simulink model "DISCON_NREL5MW_WaveFF"  (R2023b)
settings: Solver=ode1  StartTime=0.0  StopTime=inf  FixedStep=Control.TimeStep  RelTol=1e-3
InitFcn:
  | % General parameters
  | DT=0.0565685;
  | Control.TimeStep=DT;
  | gb=97;
settings Model: Creator=evansolingen  LastModifiedBy=rmojal
settings SolverCC: AlgebraicLoopSolver=TrustRegion
settings DataIOCC: LimitDataPoints=on  SaveFormat=Array  SignalLoggingSaveFormat=ModelDataLogs  SaveOutput=off  SignalLogging=off  SaveTime=off  ReturnWorkspaceOutputs=off
settings OptimizationCC: ExpressionDepthLimit=2147483647  LifeSpan=inf
settings DebuggingCC: UnderspecifiedInitializationDetection=Classic  MergeDetectMultiDrivingBlocksExec=none  SolverPrmCheckMsg=warning  MultiTaskDSMMsg=warning  MultiTaskCondExecSysMsg=none  FcnCallInpInsideContextMsg=warning  UnconnectedInputMsg=warning  UnconnectedOutputMsg=warning  UnconnectedLineMsg=warning  AllowSymbolicDim=off  StateNameClashWarn=warning  SFUnexpectedBacktrackingDiag=warning  SFNoUnconditionalDefaultTransitionDiag=warning  SFExecutionAtInitializationDiag=none  ArithmeticOperatorsInVariantConditions=warning
settings HardwareCC: ProdBitPerPointer=32  ProdBitPerSizeT=32  ProdBitPerPtrDiffT=32  ProdLargestAtomicFloat=None  ProdIntDivRoundTo=Undefined  ProdWordSize=32  ProdHWDeviceType=32-bit Generic  TargetEndianess=LittleEndian
settings ModelReferenceCC: UpdateModelReferenceTargets=Force  EnableRefExpFcnMdlSchedulingChecks=on  PropagateSignalLabelsOutOfModel=off
settings SFSimCC: SimUseLocalCustomCode=off  SimParseCustomCode=off  CustomCodeUndefinedFunction=UseInterfaceOnly
settings RTWCC: Description=DISCON DLL Target (for use with GH BLADED)  SystemTargetFile=discon.tlc  TemplateMakefile=discon.tmf  RTWUseLocalCustomCode=off
settings CodeAppCC: StateflowObjectComments=on
settings GRTTargetCC: TargetLangStandard=C89/C90 (ANSI)  CombineOutputUpdateFcns=off  GRTInterface=on  UseToolchainInfoCompliant=off  ExtModeMexFile=noextcomm
settings ConfigComp: CovMetricSettings=dw  CovSaveCumulativeToWorkspaceVar=on  CovSaveSingleToWorkspaceVar=on  CovExternalEMLEnable=off

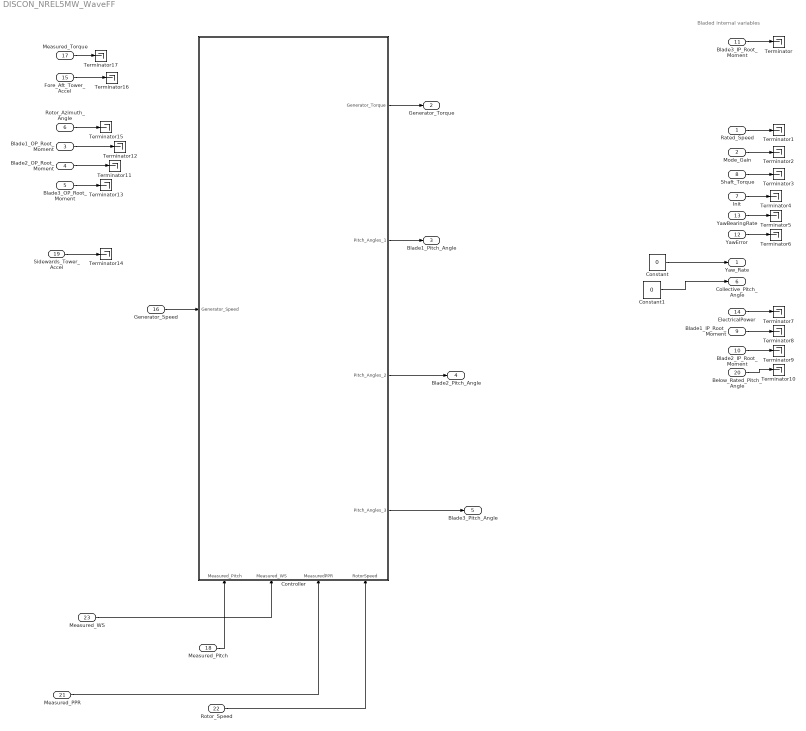
== system DISCON_NREL5MW_WaveFF ==
  note: Bladed internal variables
  Rated_Speed : Inport  PortDimensions=1
  Mode_Gain : Inport  Port=2  PortDimensions=1
  Blade1_OP_Root_Moment : Inport  Port=3  PortDimensions=1
  Blade2_OP_Root_Moment : Inport  Port=4  PortDimensions=1
  Blade3_OP_Root_Moment : Inport  Port=5  PortDimensions=1
  Rotor_Azimuth_Angle : Inport  Port=6  PortDimensions=1
  Init : Inport  Port=7  PortDimensions=1
  Shaft_Torque : Inport  Port=8  PortDimensions=1
  Blade1_IP_Root_Moment : Inport  Port=9  PortDimensions=1
  Blade2_IP_Root_Moment : Inport  Port=10  PortDimensions=1
  Blade3_IP_Root_Moment : Inport  Port=11  PortDimensions=1
  YawError : Inport  Port=12  PortDimensions=1
  YawBearingRate : Inport  Port=13  PortDimensions=1
  ElectricalPower : Inport  Port=14  PortDimensions=1
  Fore_Aft_Tower_Accel : Inport  Port=15  PortDimensions=1
  Generator_Speed : Inport  Port=16  PortDimensions=1
  Measured_Torque : Inport  Port=17  PortDimensions=1
  Measured_Pitch : Inport  Port=18  PortDimensions=1
  Sidewards_Tower_Accel : Inport  Port=19  PortDimensions=1
  Below_Rated_Pitch_Angle : Inport  Port=20  PortDimensions=1
  Measured_PPR : Inport  Port=21  PortDimensions=1
  Rotor_Speed : Inport  Port=22  PortDimensions=1
  Measured_WS : Inport  Port=23  PortDimensions=1
  Constant : Constant  Value=0
  Constant1 : Constant  Value=0
  Controller : Subsystem
      settings: PortSchema="{\"entries\":[{\"content\":{\"sides\":[{\"content\":{\"connectorIds\":[\"In1\"]},\"type\":\"ConnectorPlacement.EquallySpacedRectSide\",\"uuid\":\"5eea0745-7772-402e-b13d-af5dbe336d94\"},{\"content\":{\"connectorIds\":[\"Out1\",\"Out2\",\"Out3\",\"Out4\"],\"side\":\"RIGHT\"},\"type\":\"ConnectorPlacement.EquallySpacedRectSide\",\"uuid\":\"fe86a02a-1155-422e-9e4f-83d0aa3f1667\"},{\"content\":{\"side\":\"TOP\"},\"type\":\"ConnectorPlacement.EquallySpacedRectSide\",\"uuid\":\"d4d110c7-6a91-4408-ae2d-caf3a921c34f\"},{\"content\":{\"connectorIds\":[\"In2\",\"In3\",\"In4\",\"In5\"],\"side\":\"BOTTOM\"},\"type\":\"ConnectorPlacement.EquallySpacedRectSide\",\"uuid\":\"623fd245-908b-43aa-8a72-77a4c8000db8\"}]},\"type\":\"ConnectorPlacement.EquallySpacedConnector\",\"uuid\":\"2baef728-2889-41b2-b1a7-ad06cd068c9a\"}],\"packageUris\":[\"http://schema.mathworks.com/mf0/Connector/R2020b\"],\"version\":\"1.0\"}"
  Terminator{,1..17} (18 alike) : Terminator
  Yaw_Rate : Outport  PortDimensions=1  VectorParamsAs1DForOutWhenUnconnected=off
  Generator_Torque : Outport  Port=2  PortDimensions=1  VectorParamsAs1DForOutWhenUnconnected=off
  Blade1_Pitch_Angle : Outport  Port=3  PortDimensions=1  VectorParamsAs1DForOutWhenUnconnected=off
  Blade2_Pitch_Angle : Outport  Port=4  PortDimensions=1  VectorParamsAs1DForOutWhenUnconnected=off
  Blade3_Pitch_Angle : Outport  Port=5  PortDimensions=1  VectorParamsAs1DForOutWhenUnconnected=off
  Collective_Pitch_Angle : Outport  Port=6  PortDimensions=1  VectorParamsAs1DForOutWhenUnconnected=off
  wires:
  Generator_Speed/1 -> Controller/1(Generator_Speed)
  Controller/1(Generator_Torque) -> Generator_Torque/1
  Controller/2(Pitch_Angles_1) -> Blade1_Pitch_Angle/1
  Controller/3(Pitch_Angles_2) -> Blade2_Pitch_Angle/1
  Controller/4(Pitch_Angles_3) -> Blade3_Pitch_Angle/1
  Measured_PPR/1 -> Controller/4(MeasuredPPR)
  Rotor_Speed/1 -> Controller/5(RotorSpeed)
  Measured_WS/1 -> Controller/3(Measured_WS)
  Measured_Pitch/1 -> Controller/2(Measured_Pitch)
  Blade3_IP_Root_Moment/1 -> Terminator/1
  Rated_Speed/1 -> Terminator1/1
  Mode_Gain/1 -> Terminator2/1
  Shaft_Torque/1 -> Terminator3/1
  Init/1 -> Terminator4/1
  YawBearingRate/1 -> Terminator5/1
  YawError/1 -> Terminator6/1
  ElectricalPower/1 -> Terminator7/1
  Blade1_IP_Root_Moment/1 -> Terminator8/1
  Blade2_IP_Root_Moment/1 -> Terminator9/1
  Below_Rated_Pitch_Angle/1 -> Terminator10/1
  Blade1_OP_Root_Moment/1 -> Terminator12/1
  Blade2_OP_Root_Moment/1 -> Terminator11/1
  Blade3_OP_Root_Moment/1 -> Terminator13/1
  Sidewards_Tower_Accel/1 -> Terminator14/1
  Rotor_Azimuth_Angle/1 -> Terminator15/1
  Fore_Aft_Tower_Accel/1 -> Terminator16/1
  Measured_Torque/1 -> Terminator17/1
  Constant/1 -> Yaw_Rate/1
  Constant1/1 -> Collective_Pitch_Angle/1

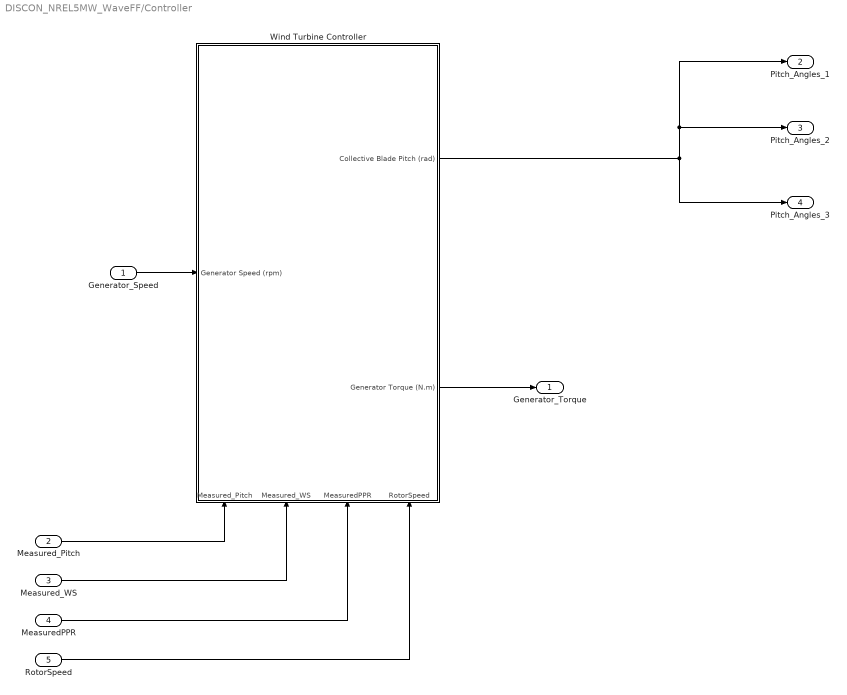
== system DISCON_NREL5MW_WaveFF/Controller ==
  Generator_Speed : Inport
  Measured_Pitch : Inport  Port=2
  Measured_WS : Inport  Port=3
  MeasuredPPR : Inport  Port=4
  RotorSpeed : Inport  Port=5
  Wind Turbine Controller : Subsystem
      settings: PortSchema="{\"entries\":[{\"content\":{\"sides\":[{\"content\":{\"connectorIds\":[\"In1\"]},\"type\":\"ConnectorPlacement.EquallySpacedRectSide\",\"uuid\":\"60e180a6-f3d9-41ac-b258-85164fa97132\"},{\"content\":{\"connectorIds\":[\"Out1\",\"Out2\"],\"side\":\"RIGHT\"},\"type\":\"ConnectorPlacement.EquallySpacedRectSide\",\"uuid\":\"a424f4c7-ff92-4106-8929-f61da2bed5ce\"},{\"content\":{\"side\":\"TOP\"},\"type\":\"ConnectorPlacement.EquallySpacedRectSide\",\"uuid\":\"4507b62c-853f-4db2-8819-247504761e25\"},{\"content\":{\"connectorIds\":[\"In2\",\"In3\",\"In4\",\"In5\"],\"side\":\"BOTTOM\"},\"type\":\"ConnectorPlacement.EquallySpacedRectSide\",\"uuid\":\"74ae92db-9457-4ead-8989-dbd06da1e1bc\"}]},\"type\":\"ConnectorPlacement.EquallySpacedConnector\",\"uuid\":\"890c16f4-d26b-446d-8a10-315b447bcdfe\"}],\"packageUris\":[\"http://schema.mathworks.com/mf0/Connector/R2020b\"],\"version\":\"1.0\"}"
  Generator_Torque : Outport  VectorParamsAs1DForOutWhenUnconnected=off
  Pitch_Angles_1 : Outport  Port=2  PortDimensions=1  VectorParamsAs1DForOutWhenUnconnected=off
  Pitch_Angles_2 : Outport  Port=3  PortDimensions=1  VectorParamsAs1DForOutWhenUnconnected=off
  Pitch_Angles_3 : Outport  Port=4  PortDimensions=1  VectorParamsAs1DForOutWhenUnconnected=off
  wires:
  Wind Turbine Controller/2(Generator Torque (N.m)) -> Generator_Torque/1
  Generator_Speed/1 -> Wind Turbine Controller/1(Generator Speed (rpm))
  Wind Turbine Controller/1(" Collective Blade Pitch (rad)") -> Pitch_Angles_1/1, Pitch_Angles_2/1, Pitch_Angles_3/1
  MeasuredPPR/1 -> Wind Turbine Controller/4(MeasuredPPR)
  RotorSpeed/1 -> Wind Turbine Controller/5(RotorSpeed)
  Measured_Pitch/1 -> Wind Turbine Controller/2(Measured_Pitch)
  Measured_WS/1 -> Wind Turbine Controller/3(Measured_WS)

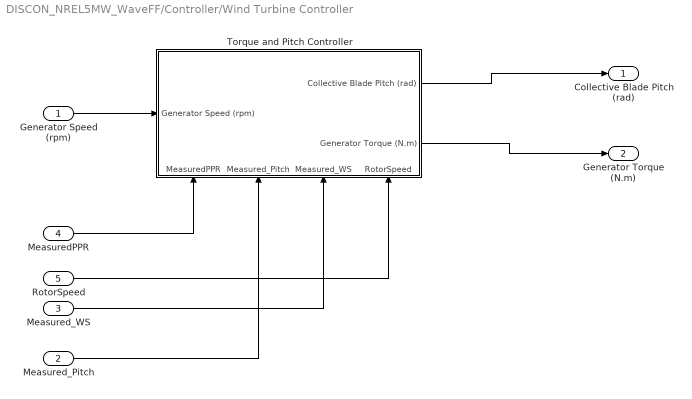
== system DISCON_NREL5MW_WaveFF/Controller/Wind Turbine Controller ==
  Generator Speed (rpm) : Inport
  Measured_Pitch : Inport  Port=2
  Measured_WS : Inport  Port=3
  MeasuredPPR : Inport  Port=4
  RotorSpeed : Inport  Port=5
  Torque and Pitch Controller : Subsystem
      settings: PortSchema="{\"entries\":[{\"content\":{\"sides\":[{\"content\":{\"connectorIds\":[\"In1\"]},\"type\":\"ConnectorPlacement.EquallySpacedRectSide\",\"uuid\":\"41f078d3-b4c7-4436-8efb-2933835bf469\"},{\"content\":{\"connectorIds\":[\"Out1\",\"Out2\"],\"side\":\"RIGHT\"},\"type\":\"ConnectorPlacement.EquallySpacedRectSide\",\"uuid\":\"44137c6d-4d2f-4b5d-90b4-72e44e418c3d\"},{\"content\":{\"side\":\"TOP\"},\"type\":\"ConnectorPlacement.EquallySpacedRectSide\",\"uuid\":\"9ef615e9-cc73-41b1-8842-e294b4be6557\"},{\"content\":{\"connectorIds\":[\"In2\",\"In3\",\"In4\",\"In5\"],\"side\":\"BOTTOM\"},\"type\":\"ConnectorPlacement.EquallySpacedRectSide\",\"uuid\":\"69c559ae-5e90-48b5-8bb5-f3e725c72204\"}]},\"type\":\"ConnectorPlacement.EquallySpacedConnector\",\"uuid\":\"6facd867-2bfd-4329-8099-ae66f4e4d363\"}],\"packageUris\":[\"http://schema.mathworks.com/mf0/Connector/R2020b\"],\"version\":\"1.0\"}"
  " Collective Blade Pitch (rad)" : Outport
  Generator Torque (N.m) : Outport  Port=2
  wires:
  Generator Speed (rpm)/1 -> Torque and Pitch Controller/1(Generator Speed (rpm))
  Torque and Pitch Controller/2(Generator Torque (N.m)) -> Generator Torque (N.m)/1
  Torque and Pitch Controller/1(" Collective Blade Pitch (rad)") -> " Collective Blade Pitch (rad)"/1
  MeasuredPPR/1 -> Torque and Pitch Controller/2(MeasuredPPR)
  RotorSpeed/1 -> Torque and Pitch Controller/5(RotorSpeed)
  Measured_WS/1 -> Torque and Pitch Controller/4(Measured_WS)
  Measured_Pitch/1 -> Torque and Pitch Controller/3(Measured_Pitch)

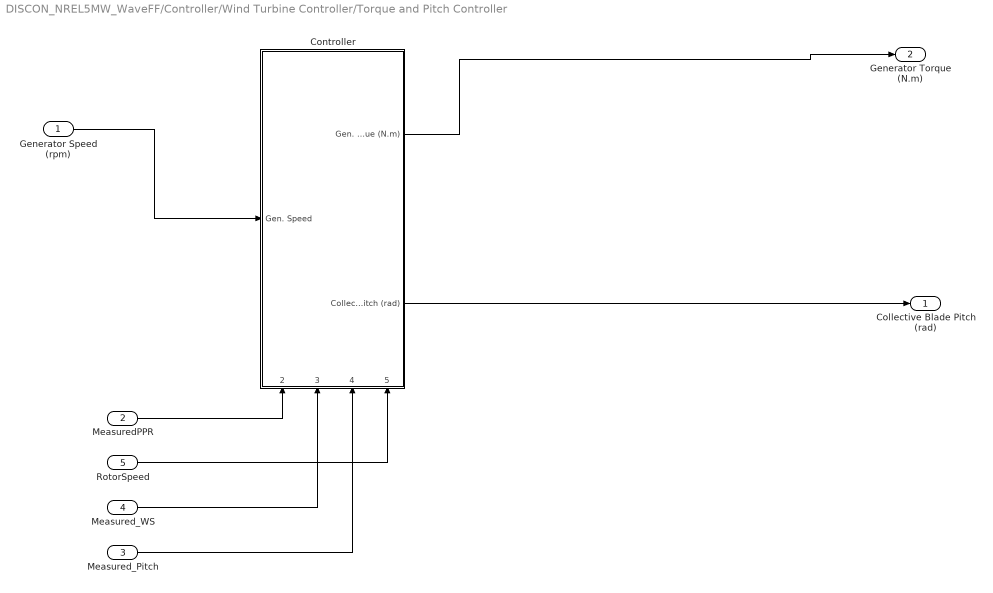
== system DISCON_NREL5MW_WaveFF/Controller/Wind Turbine Controller/Torque and Pitch Controller ==
  Generator Speed (rpm) : Inport
  MeasuredPPR : Inport  Port=2
  Measured_Pitch : Inport  Port=3
  Measured_WS : Inport  Port=4
  RotorSpeed : Inport  Port=5
  Controller : Subsystem
      settings: PortSchema="{\"entries\":[{\"content\":{\"sides\":[{\"content\":{\"connectorIds\":[\"In1\"]},\"type\":\"ConnectorPlacement.EquallySpacedRectSide\",\"uuid\":\"059e71ba-ba04-4257-a8ec-4ba8011e6b7c\"},{\"content\":{\"connectorIds\":[\"Out1\",\"Out2\"],\"side\":\"RIGHT\"},\"type\":\"ConnectorPlacement.EquallySpacedRectSide\",\"uuid\":\"7728fccf-4111-43b7-a29b-3c8202db8d59\"},{\"content\":{\"side\":\"TOP\"},\"type\":\"ConnectorPlacement.EquallySpacedRectSide\",\"uuid\":\"5cd4fe85-95f9-47fb-ae2b-ff437f261722\"},{\"content\":{\"connectorIds\":[\"In2\",\"In3\",\"In4\",\"In5\"],\"side\":\"BOTTOM\"},\"type\":\"ConnectorPlacement.EquallySpacedRectSide\",\"uuid\":\"633850b7-9343-4aec-ae47-23a99e859344\"}]},\"type\":\"ConnectorPlacement.EquallySpacedConnector\",\"uuid\":\"ea1a022b-361d-480f-a696-27bf9479e3d4\"}],\"packageUris\":[\"http://schema.mathworks.com/mf0/Connector/R2020b\"],\"version\":\"1.0\"}"
  " Collective Blade Pitch (rad)" : Outport
  Generator Torque (N.m) : Outport  Port=2
  wires:
  Controller/1(Gen. Torque (N.m)) -> Generator Torque (N.m)/1
  Generator Speed (rpm)/1 -> Controller/1(Gen. Speed)
  Controller/2(Collective Blade Pitch (rad)) -> " Collective Blade Pitch (rad)"/1
  MeasuredPPR/1 -> Controller/2(Measured_PPR)
  RotorSpeed/1 -> Controller/5(RotorSpeed)
  Measured_WS/1 -> Controller/3(Measured_WS)
  Measured_Pitch/1 -> Controller/4(Measured_Pitch)

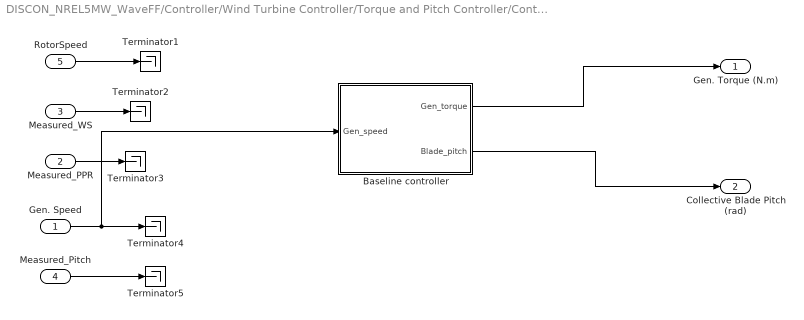
== system DISCON_NREL5MW_WaveFF/Controller/Wind Turbine Controller/Torque and Pitch Controller/Controller ==
  Gen. Speed : Inport
  Measured_PPR : Inport  Port=2
  Measured_WS : Inport  Port=3
  Measured_Pitch : Inport  Port=4
  RotorSpeed : Inport  Port=5
  Baseline controller : Subsystem
  Terminator{1..5} (5 alike) : Terminator
  Gen. Torque (N.m) : Outport
  Collective Blade Pitch (rad) : Outport  Port=2
  wires:
  RotorSpeed/1 -> Terminator1/1
  Measured_WS/1 -> Terminator2/1
  Measured_PPR/1 -> Terminator3/1
  Gen. Speed/1 -> Baseline controller/1(Gen_speed), Terminator4/1
  Measured_Pitch/1 -> Terminator5/1
  Baseline controller/1(Gen_torque) -> Gen. Torque (N.m)/1
  Baseline controller/2(Blade_pitch) -> Collective Blade Pitch (rad)/1

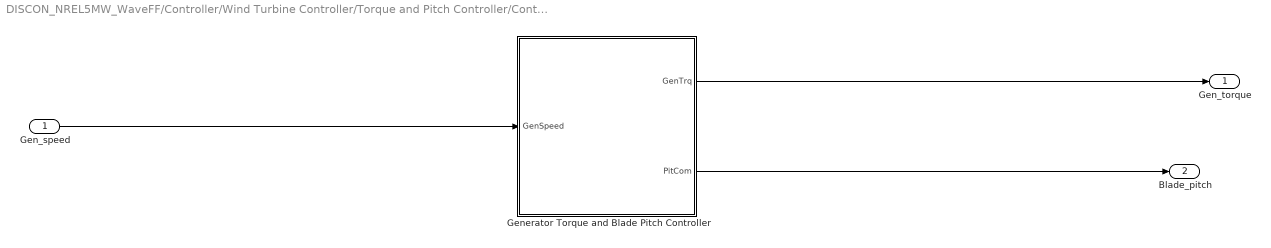
== system DISCON_NREL5MW_WaveFF/Controller/Wind Turbine Controller/Torque and Pitch Controller/Controller/Baseline controller ==
  Gen_speed : Inport
  Generator Torque and Blade Pitch Controller : MATLAB Function  TreatAsAtomicUnit=on
  Gen_torque : Outport
  Blade_pitch : Outport  Port=2
  wires:
  Generator Torque and Blade Pitch Controller/2(PitCom) -> Blade_pitch/1
  Gen_speed/1 -> Generator Torque and Blade Pitch Controller/1(GenSpeed)
  Generator Torque and Blade Pitch Controller/1(GenTrq) -> Gen_torque/1

== matlab function DISCON_NREL5MW_WaveFF/Controller/Wind Turbine Controller/Torque and Pitch Controller/Controller/Baseline controller/Generator Torque and Blade Pitch Controller ==
  data: GenTrq output; GenSpeed input; PitCom output; Control parameter
function [GenTrq, PitCom] = Controller(GenSpeed, Control)

%% Definition of the variables used in the script
% LPF_CornerFreq: Corner frequency (-3dB point) in the recursive, single-pole, low-pass filter, rad/s. -- chosen to be 1/4 the blade edgewise natural frequency ( 1/4 of approx. 1Hz = 0.25Hz = 1.570796rad/s)
% TimeStep      : Simulation time step (s)
% PC_DT         : Communication interval for pitch  controller, sec.
% PC_KI         : Integral gain for pitch controller at rated pitch (zero), (-).
% PC_KK         : Pitch angle where the the derivative of the aerodynamic power w.r.t. pitch has increased by a factor of two relative to the derivative at rated pitch (zero), rad.
% PC_KP         : Proportional gain for pitch controller at rated pitch (zero), sec.
% PC_MaxPit     : Maximum pitch setting in pitch controller, rad.
% PC_MaxRat     : Maximum pitch  rate (in absolute value) in pitch  controller, rad/s.
% PC_MinPit     : Minimum pitch setting in pitch controller, rad.
% PC_RefSpd     : Desired (reference) HSS speed for pitch controller, rad/s.
% PitCom        : Commanded pitch of each blade the last time the controller was called, rad.
% PitComI       : Integral term of command pitch, rad.
% PitComP       : Proportional term of command pitch, rad.
% PitComT       : Total command pitch based on the sum of the proportional and integral terms, rad.
% PitRate       : Pitch rates of each blade based on the current pitch angles and current pitch command, rad/s.
% SpdErr        : Current speed error, rad/s.
% TrqRate       : Torque rate based on the current and last torque commands, N-m/s.
% VS_CtInSp     : Transitional generator speed (HSS side) between regions 1 and 1 1/2, rad/s.
% VS_DT         : Communication interval for torque controller, sec.
% VS_MaxRat     : Maximum torque rate (in absolute value) in torque controller, N-m/s.
% VS_MaxTq      : Maximum generator torque in Region 3 (HSS side), N-m. -- chosen to be 10% above VS_RtTq = 43.09355kNm
% VS_Rgn2K      : Generator torque constant in Region 2 (HSS side), N-m/(rad/s)^2.
% VS_Rgn2Sp     : Transitional generator speed (HSS side) between regions 1 1/2 and 2, rad/s.
% VS_Rgn3MP     : Minimum pitch angle at which the torque is computed as if we are in region 3 regardless of the generator speed, rad. -- chosen to be 1.0 degree above PC_MinPit
% VS_RtGnSp     : Rated generator speed (HSS side), rad/s. -- chosen to be 99% of PC_RefSpd
% VS_RtPwr      : Rated generator generator power in Region 3, Watts. -- chosen to be 5MW divided by the electrical generator efficiency of 94.4%
% VS_Slope15    : Torque/speed slope of region 1 1/2 cut-in torque ramp , N-m/(rad/s).
% VS_Slope25    : Torque/speed slope of region 2 1/2 induction generator, N-m/(rad/s).
% VS_SlPc       : Rated generator slip percentage in Region 2 1/2, %.
% VS_SySp       : Synchronous speed of region 2 1/2 induction generator, rad/s.
% VS_TrGnSp     : Transitional generator speed (HSS side) between regions 2 and 2 1/2, rad/s.

% Note, each of the above variables is preceeded by the structure and the
% field where they are defined. That structure is called Control, and is
% composed of 4 field, namely, TimeStep, Filters, Torque and Pitch. 

%% Define the persistent variables in the function
persistent GenSpdFilt PitCommand GK SpdErrInt LastGenTorque 

%% Determine some torque control parameters not specified directly
VS_SySp       = Control.Torque.VS_RtGnSp/( 1.0 +  0.01*Control.Torque.VS_SlPc );                                                                         % Synchronous speed of region 2 1/2 induction generator, rad/s.
VS_Slope15    = (Control.Torque.VS_Rgn2K*Control.Torque.VS_Rgn2Sp*Control.Torque.VS_Rgn2Sp )/( Control.Torque.VS_Rgn2Sp - Control.Torque.VS_CtInSp );   % Torque/speed slope of region 1 1/2 cut-in torque ramp , N-m/(rad/s).
VS_Slope25    = ( Control.Torque.VS_RtPwr/Control.Pitch.PC_RefSpd           )/( Control.Torque.VS_RtGnSp - VS_SySp   );                                  % Torque/speed slope of region 2 1/2 induction generator , N-m/(rad/s).

if ( Control.Torque.VS_Rgn2K == 0.0 )
    VS_TrGnSp = VS_SySp;                                           % TRUE, if the torque in Region 2 is flat, and thus, the denominator in the ELSE condition is zero
else
    VS_TrGnSp = ( VS_Slope25 - sqrt( VS_Slope25*( VS_Slope25 - 4.0*Control.Torque.VS_Rgn2K*VS_SySp ) ) )/( 2.0*Control.Torque.VS_Rgn2K );
end

%% Initialize Saved Variables 
if isempty(GenSpdFilt)
    GenSpdFilt = GenSpeed;                                         % This will ensure that generator speed filter will use the initial value of the generator speed on the first pass                
    PitCommand = Control.Pitch.PC_MinPit;                          % This will ensure that the variable speed controller picks the correct control region and the pitch controller picks the correct gain on the first call
    GK         = 1.0/( 1.0 + PitCommand/Control.Pitch.PC_KK );     % This will ensure that the pitch angle is unchanged if the initial SpdErr is zero
    SpdErrInt  = PitCommand/( GK*Control.Pitch.PC_KI );            % This will ensure that the pitch angle is unchanged if the initial SpdErr is zero    
end

%% ============================= Filtering ============================= %%
% Filter the HSS (generator) speed measurement
% NOTE: This is a very simple recursive, single-pole, low-pass filter with exponential smoothing.
Alpha         = exp( -Control.TimeStep * Control.Filters.LPF_CornerFreq );

% Apply the Filter
GenSpeedF = ( 1.0 - Alpha )*GenSpeed + Alpha * GenSpdFilt;

% Update the persistent variable GenSpdFilt (This is to store the value of the presistent variable to be e used in the next time step)
GenSpdFilt = GenSpeedF;
     
%% =================== Variable-Speed Torque Control =================== %%
% Compute the generator torque, which depends on which region we are in:
if(GenSpeedF >= Control.Torque.VS_RtGnSp)||( PitCommand>= Control.Torque.VS_Rgn3MP )                   % We are in region 3 - power is constant
    GenTrq = Control.Torque.VS_RtPwr/Control.Pitch.PC_RefSpd;
elseif(GenSpeedF <= Control.Torque.VS_CtInSp)                                                          % We are in region 1 - torque is zero
    GenTrq = 0.0;
elseif(GenSpeedF <  Control.Torque.VS_Rgn2Sp)                                                          % We are in region 1 1/2 - linear ramp in torque from zero to optimal
    GenTrq = VS_Slope15*( GenSpeedF - Control.Torque.VS_CtInSp );
elseif(GenSpeedF <  VS_TrGnSp)                                                                         % We are in region 2 - optimal torque is proportional to the square of the generator speed
    GenTrq = Control.Torque.VS_Rgn2K*GenSpeedF*GenSpeedF;
else                                                                                                   % We are in region 2 1/2 - simple induction generator transition region
    GenTrq = VS_Slope25*( GenSpeedF - VS_SySp   );
end

% Saturate the commanded torque using the maximum torque limit:
GenTrq  = min( GenTrq, Control.Torque.VS_MaxTq  );                                                     % Saturate the command using the maximum torque limit

% Saturate the commanded torque using the torque rate limit:
if isempty(LastGenTorque)
    LastGenTorque = GenTrq;                                                                            % Initialize the value of LastGenTrq on the first pass only
end

TrqRate = ( GenTrq - LastGenTorque )/Control.TimeStep;                                                 % Torque rate (unsaturated)         
TrqRate = min( max( TrqRate, -Control.Torque.VS_MaxRat ), Control.Torque.VS_MaxRat );                  % Saturate the torque rate using its maximum absolute value
GenTrq  = LastGenTorque + TrqRate*Control.TimeStep;                                                    % Saturate the command using the torque rate limit

% Store the value of LastGenTorque for the next time step:
LastGenTorque = GenTrq;


%% =========================== Pitch Control =========================== %%

% Compute the gain scheduling correction factor based on the previously commanded pitch angle for blade 1:
GK = 1.0/( 1.0 + PitCommand/Control.Pitch.PC_KK );                    

% Compute the current speed error and its integral w.r.t. time;
% saturate the integral term using the pitch angle limits:
SpdErr    = GenSpdFilt - Control.Pitch.PC_RefSpd;                                                     % Current speed error        
IntSpdErr = SpdErrInt + SpdErr*Control.TimeStep;                                                      % Current integral of speed error w.r.t. time             
IntSpdErr = min( max( IntSpdErr, Control.Pitch.PC_MinPit/( GK*Control.Pitch.PC_KI ) ), Control.Pitch. PC_MaxPit/( GK*Control.Pitch.PC_KI ));    % Saturate the integral term using the pitch angle limits, converted to integral speed error limits

% Compute the pitch commands associated with the proportional and integral gains:
PitComP   = GK*Control.Pitch.PC_KP*SpdErr;                                                            % Proportional term          
PitComI   = GK*Control.Pitch.PC_KI*IntSpdErr;                                                         % Integral term (saturated) 

% Superimpose the individual commands to get the total pitch command;
%  saturate the overall command using the pitch angle limits:
PitComT   = PitComP + PitComI;                                                                        % Overall command (unsaturated)       
PitComT   = min( max( PitComT, Control.Pitch.PC_MinPit ), Control.Pitch.PC_MaxPit );                  % Saturate the overall command using the pitch angle limits

% Saturate the overall commanded pitch using the pitch rate limit:
% NOTE: Since the current pitch angle may be different for each blade
% (depending on the type of actuator implemented in the structural
% dynamics model), this pitch rate limit calculation and the 
% resulting overall pitch angle command may be different for each blade.
PitRate   = ( PitComT - PitCommand)/Control.TimeStep;                                                 % Pitch rate of the blades (unsaturated)           
PitRate   = min( max( PitRate, -Control.Pitch.PC_MaxRat ), Control.Pitch.PC_MaxRat );                 % Saturate the pitch rate of the blade using its maximum absolute value

PitCom    = PitCommand + PitRate*Control.TimeStep;                                                    % Saturate the overall command of the blade using the pitch rate limit           
PitCom    = min( max( PitCom, Control.Pitch.PC_MinPit ), Control.Pitch.PC_MaxPit );                   % Saturate the overall command using the pitch angle limits

% Store the persistent variables to be used in the next time step)
PitCommand = PitCom;
SpdErrInt = IntSpdErr;
